simulink library "LM_LIB"  (R2019b)
settings: Solver=VariableStepAuto  StartTime=0.0  StopTime=10.0  RelTol=1e-3
undefined symbols (not defined in the file): P_LM_FusBLParFiltP, P_LM_FusParC0Index, P_LM_FusParC1Index, P_LM_FusParC2Index, P_LM_FusParC3Index, P_LM_OTLBufTPMinPntNum, P_LM_OTLBufTPSPosMinDis, P_LM_OTLRearMaxDis, P_LM_OTLTPNum
libraries: simulink x84, $bdroot x3
(part 2 of 5)

== system LM_LIB/LM_LineInfo1/LM_Line_Fnt ==
  LM_LineC0 : Inport
  LM_PathDisBus : Inport  Port=2
  LM_FusBLInfoFilt : Inport  Port=3
  LM_FusfCamValidInfo : Inport  Port=4
  Bus Selector1 : BusSelector  OutputSignals=LM_FntPath1Dis
  Bus Selector10 : BusSelector  OutputSignals=LM_FusBLFntPath1Info.LM_FusBLPathC0,LM_FusBLFntPath1Info.LM_FusBLPathC1,LM_FusBLFntPath1Info.LM_FusBLPathC2,LM_FusBLFntPath1Info.LM_FusBLPathC3,LM_FusBLFntPath1Info.LM_FusBLPathQuality
  Bus Selector2 : BusSelector  OutputSignals=LM_FntPath1Dis,LM_FntPath2Dis
  Bus Selector3 : BusSelector  OutputSignals=LM_FusBLFntPath2Info.LM_FusBLPathC0,LM_FusBLFntPath2Info.LM_FusBLPathC1,LM_FusBLFntPath2Info.LM_FusBLPathC2,LM_FusBLFntPath2Info.LM_FusBLPathC3,LM_FusBLFntPath2Info.LM_FusBLPathQuality
  Bus Selector5 : BusSelector  OutputSignals=LM_FntPath2Dis,LM_FntPath3Dis
  Bus Selector6 : BusSelector  OutputSignals=LM_FusBLFntPath3Info.LM_FusBLPathC0,LM_FusBLFntPath3Info.LM_FusBLPathC1,LM_FusBLFntPath3Info.LM_FusBLPathC2,LM_FusBLFntPath3Info.LM_FusBLPathC3,LM_FusBLFntPath3Info.LM_FusBLPathQuality
  Bus Selector7 : BusSelector  OutputSignals=LM_FusFntPath1fCamValid
  Bus Selector8 : BusSelector  OutputSignals=LM_FusFntPath2fCamValid
  Bus Selector9 : BusSelector  OutputSignals=LM_FusFntPath3fCamValid
  LM_Path04 : Subsystem
  LM_Path05 : Subsystem
  LM_Path06 : Subsystem
  LM_Path07 : Subsystem
  LM_Path08 : Subsystem
  LM_Line04 : Outport
  LM_Line05 : Outport  Port=2
  LM_LL_Line06 : Outport  Port=3
  LM_LL_Line07 : Outport  Port=4
  LM_LL_Line08 : Outport  Port=5
  wires:
  Bus Selector6/1 -> LM_Path06/2(LM_FusBLFntPath3C0)  "<LM_FusBLPathC0>"
  Bus Selector6/5 -> LM_Path06/6(LM_FusBLFntPath3Quality)  "<LM_FusBLPathQuality>"
  Bus Selector6/4 -> LM_Path06/5(LM_FusBLFntPath3C3)  "<LM_FusBLPathC3>"
  Bus Selector6/3 -> LM_Path06/4(LM_FusBLFntPath3C2)  "<LM_FusBLPathC2>"
  Bus Selector6/2 -> LM_Path06/3(LM_FusBLFntPath3C1)  "<LM_FusBLPathC1>"
  Bus Selector3/1 -> LM_Path05/3(LM_FusBLFntPath2C0)  "<LM_FusBLPathC0>"
  Bus Selector3/5 -> LM_Path05/7(LM_FusBLFntPath2Quality)  "<LM_FusBLPathQuality>"
  Bus Selector3/4 -> LM_Path05/6(LM_FusBLFntPath2C3)  "<LM_FusBLPathC3>"
  Bus Selector3/3 -> LM_Path05/5(LM_FusBLFntPath2C2)  "<LM_FusBLPathC2>"
  Bus Selector3/2 -> LM_Path05/4(LM_FusBLFntPath2C1)  "<LM_FusBLPathC1>"
  Bus Selector10/1 -> LM_Path04/1(LM_FusBLFntPath1C0)  "<LM_FusBLPathC0>"
  Bus Selector10/5 -> LM_Path04/5(LM_FusBLFntPath1Quality)  "<LM_FusBLPathQuality>"
  Bus Selector10/4 -> LM_Path04/4(LM_FusBLFntPath1C3)  "<LM_FusBLPathC3>"
  Bus Selector10/3 -> LM_Path04/3(LM_FusBLFntPath1C2)  "<LM_FusBLPathC2>"
  Bus Selector10/2 -> LM_Path04/2(LM_FusBLFntPath1C1)  "<LM_FusBLPathC1>"
  LM_Path07/1(LM_Line07) -> LM_LL_Line07/1
  LM_Path08/1(LM_Line08) -> LM_LL_Line08/1
  LM_Path06/1(LM_Line06) -> LM_LL_Line06/1
  LM_Path05/1(LM_Line05) -> LM_Line05/1
  LM_Path04/1(LM_Line04) -> LM_Line04/1
  Bus Selector5/2 -> LM_Path06/8(LM_FusBLFntPath3Dis)  "<LM_FntPath3Dis>"
  Bus Selector5/1 -> LM_Path06/7(LM_FusBLFntPath2Dis)  "<LM_FntPath2Dis>"
  LM_LineC0/1 -> LM_Path06/1(LM_LineC0), LM_Path05/8(LM_LineC0), LM_Path04/6(LM_LineC0)
  LM_FusBLInfoFilt/1 -> Bus Selector10/1, Bus Selector6/1, Bus Selector3/1
  Bus Selector2/1 -> LM_Path05/1(LM_FusFntPath1Dis)  "<LM_FntPath1Dis>"
  Bus Selector2/2 -> LM_Path05/2(LM_FusFntPath2Dis)  "<LM_FntPath2Dis>"
  Bus Selector1/1 -> LM_Path04/7(LM_FusFntPath1Dis)  "<LM_FntPath1Dis>"
  LM_PathDisBus/1 -> Bus Selector1/1, Bus Selector5/1, Bus Selector2/1
  LM_FusfCamValidInfo/1 -> Bus Selector7/1, Bus Selector8/1, Bus Selector9/1
  Bus Selector7/1 -> LM_Path04/8(LM_FusFntPath1fCamValid)  "<LM_FusFntPath1fCamValid>"
  Bus Selector8/1 -> LM_Path05/9(LM_FusFntPath2fCamValid)  "<LM_FusFntPath2fCamValid>"
  Bus Selector9/1 -> LM_Path06/9(LM_FusFntPath3fCamValid)  "<LM_FusFntPath3fCamValid>"

== system LM_LIB/LM_LineInfo1/LM_Line_Rear ==
  LM_FusBLInfoFilt : Inport
  LM_PathDisBus : Inport  Port=2
  LM_LineC0 : Inport  Port=3
  Bus Selector1 : BusSelector  OutputSignals=LM_RearPath1Dis
  Bus Selector10 : BusSelector  OutputSignals=LM_RearPath2Dis,LM_RearPath3Dis
  Bus Selector2 : BusSelector  OutputSignals=LM_FusBLRearPath2Info.LM_FusBLPathC0,LM_FusBLRearPath2Info.LM_FusBLPathC1,LM_FusBLRearPath2Info.LM_FusBLPathC2,LM_FusBLRearPath2Info.LM_FusBLPathC3,LM_FusBLRearPath2Info.LM_FusBLPathQuality
  Bus Selector3 : BusSelector  OutputSignals=LM_FusBLRearPath3Info.LM_FusBLPathC0,LM_FusBLRearPath3Info.LM_FusBLPathC1,LM_FusBLRearPath3Info.LM_FusBLPathC2,LM_FusBLRearPath3Info.LM_FusBLPathC3,LM_FusBLRearPath3Info.LM_FusBLPathQuality
  Bus Selector6 : BusSelector  OutputSignals=LM_FusBLRearPath1Info.LM_FusBLPathC0,LM_FusBLRearPath1Info.LM_FusBLPathC1,LM_FusBLRearPath1Info.LM_FusBLPathC2,LM_FusBLRearPath1Info.LM_FusBLPathC3,LM_FusBLRearPath1Info.LM_FusBLPathQuality
  Bus Selector8 : BusSelector  OutputSignals=LM_RearPath1Dis,LM_RearPath2Dis
  LM_Path01 : Subsystem
  LM_Path02 : Subsystem
  LM_Path03 : Subsystem
  LM_Line01 : Outport
  LM_Line02 : Outport  Port=2
  LM_Line03 : Outport  Port=3
  wires:
  Bus Selector10/2 -> LM_Path01/8(LM_RearPath3Dis)  "<LM_RearPath3Dis>"
  Bus Selector10/1 -> LM_Path01/7(LM_RearPath12Dis)  "<LM_RearPath2Dis>"
  Bus Selector3/5 -> LM_Path01/5(LM_FusBLRearPath3Quality)  "<LM_FusBLPathQuality>"
  Bus Selector3/4 -> LM_Path01/4(LM_FusBLRearPath3C3)  "<LM_FusBLPathC3>"
  Bus Selector3/3 -> LM_Path01/3(LM_FusBLRearPath3C2)  "<LM_FusBLPathC2>"
  Bus Selector3/2 -> LM_Path01/2(LM_FusBLRearPath3C1)  "<LM_FusBLPathC1>"
  Bus Selector3/1 -> LM_Path01/1(LM_FusBLRearPath3C0)  "<LM_FusBLPathC0>"
  LM_Path02/1(LM_Line02) -> LM_Line02/1
  Bus Selector8/2 -> LM_Path02/8(LM_RearPath2Dis)  "<LM_RearPath2Dis>"
  Bus Selector8/1 -> LM_Path02/7(LM_RearPath1Dis)  "<LM_RearPath1Dis>"
  Bus Selector2/5 -> LM_Path02/5(LM_FusBLRearPath2Quality)  "<LM_FusBLPathQuality>"
  Bus Selector2/4 -> LM_Path02/4(LM_FusBLRearPath2C3)  "<LM_FusBLPathC3>"
  Bus Selector2/3 -> LM_Path02/3(LM_FusBLRearPath2C2)  "<LM_FusBLPathC2>"
  Bus Selector2/2 -> LM_Path02/2(LM_FusBLRearPath2C1)  "<LM_FusBLPathC1>"
  Bus Selector2/1 -> LM_Path02/1(LM_FusBLRearPath2C0)  "<LM_FusBLPathC0>"
  Bus Selector6/1 -> LM_Path03/1(LM_FusBLRearPath1C0)  "<LM_FusBLPathC0>"
  Bus Selector6/2 -> LM_Path03/2(LM_FusBLRearPath1C1)  "<LM_FusBLPathC1>"
  Bus Selector6/5 -> LM_Path03/5(LM_FusBLRearPath1Quality)  "<LM_FusBLPathQuality>"
  Bus Selector6/3 -> LM_Path03/3(LM_FusBLRearPath1C2)  "<LM_FusBLPathC2>"
  Bus Selector6/4 -> LM_Path03/4(LM_FusBLRearPath1C3)  "<LM_FusBLPathC3>"
  LM_FusBLInfoFilt/1 -> Bus Selector6/1, Bus Selector3/1, Bus Selector2/1
  LM_PathDisBus/1 -> Bus Selector1/1, Bus Selector8/1, Bus Selector10/1
  Bus Selector1/1 -> LM_Path03/7(LM_RearPath1Dis)  "<LM_RearPath1Dis>"
  LM_LineC0/1 -> LM_Path01/6(LM_LineC0), LM_Path02/6(LM_LineC0), LM_Path03/6(LM_LineC0)
  LM_Path03/1(LM_Line03) -> LM_Line03/1
  LM_Path01/1(LM_Line01) -> LM_Line01/1

== system LM_LIB/LM_OTLBuf1InfoNew/LM_OTL_BufLe1InfoUpdate ==
  LM_OTLBufL1DxVectK1Adju : Inport
  LM_OTLBufL1DyVectK1Adju : Inport  Port=2
  LM_OTLBufL1UpdateFlg : Inport  Port=3
  LM_OTLBufL1Objdx : Inport  Port=4
  LM_OTLBufL1Objdy : Inport  Port=5
  LM_OTLBufL1EPPos : Inport  Port=6
  If : If  IfExpression=u1 ~= 0
  If Action Subsystem : Subsystem  TreatAsAtomicUnit=on
  If Action Subsystem1 : Subsystem  TreatAsAtomicUnit=on
  Merge : Merge
  Merge1 : Merge
  LM_OTLBufL1DxVect : Outport  OutDataTypeStr=single  PortDimensions=80
  LM_OTLBufL1DyVect : Outport  Port=2  OutDataTypeStr=single  PortDimensions=80
  wires:
  Merge1/1 -> LM_OTLBufL1DyVect/1  "LM_OTLBufL1DyVect"
  If Action Subsystem1/2(LM_OTLBufL1DyVect) -> Merge1/2
  If Action Subsystem/2(LM_OTLBufL1DyVect) -> Merge1/1
  Merge/1 -> LM_OTLBufL1DxVect/1  "LM_OTLBufL1DxVect"
  If Action Subsystem1/1(LM_OTLBufL1DxVect) -> Merge/2
  If Action Subsystem/1(LM_OTLBufL1DxVect) -> Merge/1
  LM_OTLBufL1EPPos/1 -> If Action Subsystem/3(LM_OTLBufL1EPPos)
  LM_OTLBufL1Objdy/1 -> If Action Subsystem/2(LM_OTLBufL1Objdy)
  LM_OTLBufL1Objdx/1 -> If Action Subsystem/1(LM_OTLBufL1Objdx)
  LM_OTLBufL1DyVectK1Adju/1 -> If Action Subsystem1/2(LM_OTLBufL1DyVectK1Adju), If Action Subsystem/5(LM_OTLBufL1DyVectK1Adju)
  LM_OTLBufL1DxVectK1Adju/1 -> If Action Subsystem1/1(LM_OTLBufL1DxVectK1Adju), If Action Subsystem/4(LM_OTLBufL1DxVectK1Adju)
  If/2 -> If Action Subsystem1/Action
  If/1 -> If Action Subsystem/Action
  LM_OTLBufL1UpdateFlg/1 -> If/1

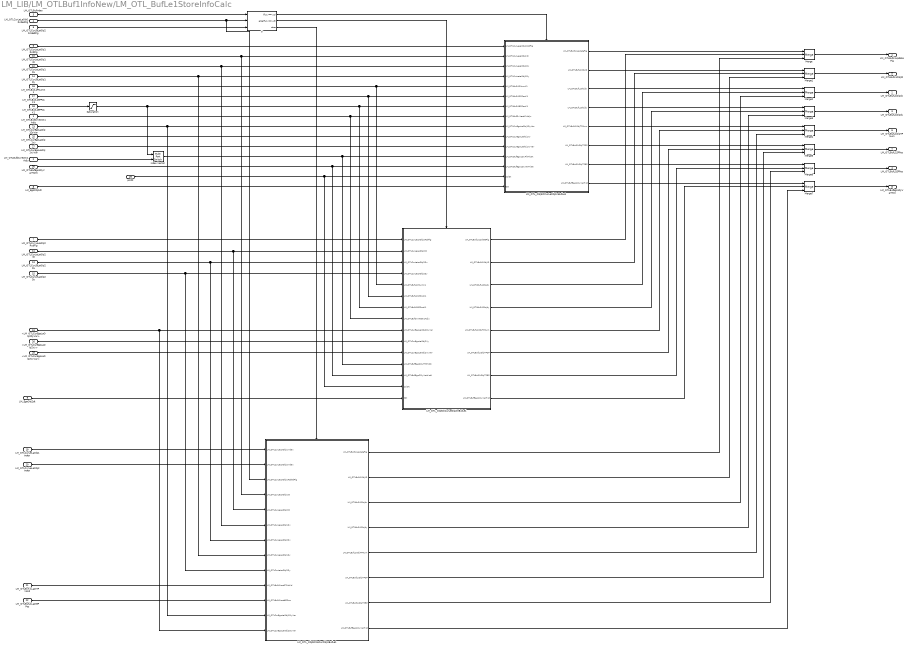
== system LM_LIB/LM_OTLBuf1InfoNew/LM_OTL_BufLe1StoreInfoCalc ==
  LM_OTLBufDxVectK1Adju : Inport
  LM_OTLBufDyVectK1Adju : Inport  Port=2
  LM_OTLBufIndex : Inport  Port=3
  LM_OTLCurLeLaObj1RcdedFlg : Inport  Port=4
  LM_OTLCurLeLaObj2RcdedFlg : Inport  Port=5
  LM_OTLCurLeLaObj1RcdFlg : Inport  Port=6
  LM_OTLCurLeLaObj2RcdFlg : Inport  Port=7
  LM_EgoObj1dt : Inport  Port=8
  LM_EgoObj2dt : Inport  Port=9
  LM_OTLCurLeLaObj1ID : Inport  Port=10
  LM_OTLCurLeLaObj2ID : Inport  Port=11
  LM_OTLCurLeLaObj1Dx : Inport  Port=12
  LM_OTLCurLeLaObj2Dx : Inport  Port=13
  LM_OTLCurLeLaObj1Dy : Inport  Port=14
  LM_OTLCurLeLaObj2Dy : Inport  Port=15
  LM_OTLBufL1PNumK1 : Inport  Port=16
  LM_OTLBufL1SPPosK1 : Inport  Port=17
  LM_OTLBufL1EPPosK1 : Inport  Port=18
  LM_OTLCurLeLaObj1Index : Inport  Port=19
  LM_OTLCurLeLaObj2Index : Inport  Port=20
  LM_OTLBufL1LastTPValid : Inport  Port=21
  LM_OTLBufL1LastEPPos : Inport  Port=22
  LM_OTLCurEgoLaObj1DyVar : Inport  Port=23
  <LM_OTLCurEgoLaObj2DyVar> : Inport  Port=24
  LM_OTLCurEgoLaObj1Vy : Inport  Port=25
  <LM_OTLCurEgoLaObj2Vy> : Inport  Port=26
  LM_OTLCurEgoLaObj1VyVar : Inport  Port=27
  <LM_OTLCurEgoLaObj2VyVar> : Inport  Port=28
  psiDt : Inport  Port=29
  LM_OTLBufEgo1DyVarHistK : Inport  Port=30
  If : If  NumInputs=3  IfExpression=u1 == u2  ElseIfExpressions=u1 == u3
  Index Vector : MultiPortSwitch  Inputs=1
  LM_OTL_ObjSICCurLeObj1InBufLe1 : Subsystem
  LM_OTL_ObjSICCurLeObj2InBufLe1 : Subsystem
  LM_OTL_ObjSICNoCurObjInBufLe1 : Subsystem
  Merge{,1..7} (8 alike) : Merge  Inputs=3
  Saturation : Saturate  UpperLimit=80  LowerLimit=1
  LM_OTLBufL1UpdateFlg : Outport
  LM_OTLBufL1Objdx : Outport  Port=2
  LM_OTLBufL1Objdy : Outport  Port=3
  LM_OTLBufL1EPPos : Outport  Port=4
  LM_OTLBufL1ObjID : Outport  Port=5
  LM_OTLBufL1ObjTPNum : Outport  Port=6
  LM_OTLBufL1SPPos : Outport  Port=7
  LM_OTLBufEgo1DyVarHist : Outport  Port=8
  wires:
  LM_OTLBufIndex/1 -> If/1
  If/1 -> LM_OTL_ObjSICCurLeObj1InBufLe1/Action
  If/2 -> LM_OTL_ObjSICCurLeObj2InBufLe1/Action
  If/3 -> LM_OTL_ObjSICNoCurObjInBufLe1/Action
  LM_OTLCurLeLaObj1RcdedFlg/1 -> If/2, LM_OTL_ObjSICNoCurObjInBufLe1/3(LM_OTLCurLeLaObj1RcdedFlg)
  LM_OTLCurLeLaObj2RcdedFlg/1 -> If/3
  LM_OTLCurLeLaObj1RcdFlg/1 -> LM_OTL_ObjSICCurLeObj1InBufLe1/1(LM_OTLCurLeLaObj1RcdFlg)
  LM_OTLCurLeLaObj1ID/1 -> LM_OTL_ObjSICNoCurObjInBufLe1/4(LM_OTLCurLeLaObj1ID), LM_OTL_ObjSICCurLeObj1InBufLe1/2(LM_OTLCurLeLaObj1ID)
  LM_OTLCurLeLaObj1Dx/1 -> LM_OTL_ObjSICCurLeObj1InBufLe1/3(LM_OTLCurLeLaObj1Dx), LM_OTL_ObjSICNoCurObjInBufLe1/6(LM_OTLCurLeLaObj1Dx)
  LM_OTLCurLeLaObj1Dy/1 -> LM_OTL_ObjSICCurLeObj1InBufLe1/4(LM_OTLCurLeLaObj1Dy), LM_OTL_ObjSICNoCurObjInBufLe1/8(LM_OTLCurLeLaObj1Dy)
  LM_OTLBufL1PNumK1/1 -> LM_OTL_ObjSICCurLeObj2InBufLe1/5(LM_OTLBufL1PNumK1), LM_OTL_ObjSICCurLeObj1InBufLe1/5(LM_OTLBufL1PNumK1)
  LM_OTLBufL1SPPosK1/1 -> LM_OTL_ObjSICCurLeObj2InBufLe1/6(LM_OTLBufL1SPPosK1), LM_OTL_ObjSICCurLeObj1InBufLe1/6(LM_OTLBufL1SPPosK1)
  LM_OTLBufL1EPPosK1/1 -> Saturation/1
  LM_OTLCurLeLaObj2RcdFlg/1 -> LM_OTL_ObjSICCurLeObj2InBufLe1/1(LM_OTLCurLeLaObj2RcdFlg)
  LM_OTLCurLeLaObj2ID/1 -> LM_OTL_ObjSICNoCurObjInBufLe1/5(LM_OTLCurLeLaObj2ID), LM_OTL_ObjSICCurLeObj2InBufLe1/2(LM_OTLCurLeLaObj2ID)
  LM_OTLCurLeLaObj2Dx/1 -> LM_OTL_ObjSICNoCurObjInBufLe1/7(LM_OTLCurLeLaObj2Dx), LM_OTL_ObjSICCurLeObj2InBufLe1/3(LM_OTLCurLeLaObj2Dx)
  LM_OTLCurLeLaObj2Dy/1 -> LM_OTL_ObjSICNoCurObjInBufLe1/9(LM_OTLCurLeLaObj2Dy), LM_OTL_ObjSICCurLeObj2InBufLe1/4(LM_OTLCurLeLaObj2Dy)
  Merge/1 -> LM_OTLBufL1UpdateFlg/1
  Merge1/1 -> LM_OTLBufL1ObjID/1
  Merge2/1 -> LM_OTLBufL1Objdx/1
  Merge3/1 -> LM_OTLBufL1Objdy/1
  Merge4/1 -> LM_OTLBufL1ObjTPNum/1
  Merge5/1 -> LM_OTLBufL1SPPos/1
  LM_OTLCurLeLaObj1Index/1 -> LM_OTL_ObjSICNoCurObjInBufLe1/1(LM_OTLCurLeLaObj1Index)
  LM_OTLCurLeLaObj2Index/1 -> LM_OTL_ObjSICNoCurObjInBufLe1/2(LM_OTLCurLeLaObj2Index)
  LM_OTLBufL1LastTPValid/1 -> LM_OTL_ObjSICNoCurObjInBufLe1/10(LM_OTLBufL1LastTPValid)
  LM_OTLBufL1LastEPPos/1 -> LM_OTL_ObjSICNoCurObjInBufLe1/11(LM_OTLBufL1LastEPPos)
  LM_OTLBufDxVectK1Adju/1 -> LM_OTL_ObjSICCurLeObj2InBufLe1/8(LM_OTLBufDxVectK1Adju), LM_OTL_ObjSICCurLeObj1InBufLe1/8(LM_OTLBufDxVectK1Adju)
  LM_OTLCurEgoLaObj1DyVar/1 -> LM_OTL_ObjSICCurLeObj1InBufLe1/9(LM_OTLCurEgoLaObj1DyVar), LM_OTL_ObjSICNoCurObjInBufLe1/12(LM_OTLCurEgoLaObj1DyVar)
  LM_OTLCurEgoLaObj1Vy/1 -> LM_OTL_ObjSICCurLeObj1InBufLe1/10(LM_OTLCurEgoLaObj1Vy)
  LM_OTLCurEgoLaObj1VyVar/1 -> LM_OTL_ObjSICCurLeObj1InBufLe1/11(LM_OTLCurEgoLaObj1VyVar)
  LM_OTLBufEgo1DyVarHistK/1 -> LM_OTL_ObjSICCurLeObj2InBufLe1/13(LM_OTLBufEgo2DyVarHistK), LM_OTL_ObjSICCurLeObj1InBufLe1/13(LM_OTLBufEgo1DyVarHistK)
  LM_OTLBufDyVectK1Adju/1 -> Index Vector/2
  Index Vector/1 -> LM_OTL_ObjSICCurLeObj2InBufLe1/12(LM_OTLBufEgo2DyFiltHistK), LM_OTL_ObjSICCurLeObj1InBufLe1/12(LM_OTLBufEgo1DyFiltHistK)
  LM_EgoObj1dt/1 -> LM_OTL_ObjSICCurLeObj1InBufLe1/15(tDt)
  psiDt/1 -> LM_OTL_ObjSICCurLeObj2InBufLe1/14(psiDt), LM_OTL_ObjSICCurLeObj1InBufLe1/14(psiDt)
  LM_EgoObj2dt/1 -> LM_OTL_ObjSICCurLeObj2InBufLe1/15(tDt)
  <LM_OTLCurEgoLaObj2DyVar>/1 -> LM_OTL_ObjSICNoCurObjInBufLe1/13(LM_OTLCurEgoLaObj2DyVar), LM_OTL_ObjSICCurLeObj2InBufLe1/9(LM_OTLCurEgoLaObj2DyVar)
  <LM_OTLCurEgoLaObj2Vy>/1 -> LM_OTL_ObjSICCurLeObj2InBufLe1/10(LM_OTLCurEgoLaObj2Vy)
  <LM_OTLCurEgoLaObj2VyVar>/1 -> LM_OTL_ObjSICCurLeObj2InBufLe1/11(LM_OTLCurEgoLaObj2VyVar)
  LM_OTL_ObjSICCurLeObj1InBufLe1/2(LM_OTLBufL1ObjID) -> Merge1/1
  LM_OTL_ObjSICCurLeObj1InBufLe1/3(LM_OTLBufL1Objdx) -> Merge2/1
  LM_OTL_ObjSICCurLeObj1InBufLe1/1(LM_OTLBufL1UpdateFlg) -> Merge/1
  LM_OTL_ObjSICCurLeObj1InBufLe1/4(LM_OTLBufL1Objdy) -> Merge3/1
  LM_OTL_ObjSICCurLeObj1InBufLe1/5(LM_OTLBufL1ObjTPNum) -> Merge4/1
  LM_OTL_ObjSICCurLeObj1InBufLe1/6(LM_OTLBufL1ObjTPSP) -> Merge5/1
  LM_OTL_ObjSICCurLeObj1InBufLe1/7(LM_OTLBufL1ObjTPEP) -> Merge6/1
  LM_OTL_ObjSICCurLeObj2InBufLe1/1(LM_OTLBufL1UpdateFlg) -> Merge/2
  LM_OTL_ObjSICCurLeObj2InBufLe1/2(LM_OTLBufL1ObjID) -> Merge1/2
  LM_OTL_ObjSICCurLeObj2InBufLe1/3(LM_OTLBufL1Objdx) -> Merge2/2
  LM_OTL_ObjSICCurLeObj2InBufLe1/4(LM_OTLBufL1Objdy) -> Merge3/2
  LM_OTL_ObjSICCurLeObj2InBufLe1/5(LM_OTLBufL1ObjTPNum) -> Merge4/2
  LM_OTL_ObjSICCurLeObj2InBufLe1/6(LM_OTLBufL1ObjTPSP) -> Merge5/2
  LM_OTL_ObjSICCurLeObj2InBufLe1/7(LM_OTLBufL1ObjTPEP) -> Merge6/2
  LM_OTL_ObjSICCurLeObj1InBufLe1/8(LM_OTLBufEgo1DyVarHist) -> Merge7/1
  Merge6/1 -> LM_OTLBufL1EPPos/1
  Merge7/1 -> LM_OTLBufEgo1DyVarHist/1
  LM_OTL_ObjSICCurLeObj2InBufLe1/8(LM_OTLBufEgo1DyVarHist) -> Merge7/2
  LM_OTL_ObjSICNoCurObjInBufLe1/1(LM_OTLBufL1UpdateFlg) -> Merge/3
  LM_OTL_ObjSICNoCurObjInBufLe1/2(LM_OTLBufL1ObjID) -> Merge1/3
  LM_OTL_ObjSICNoCurObjInBufLe1/3(LM_OTLBufL1Objdx) -> Merge2/3
  LM_OTL_ObjSICNoCurObjInBufLe1/4(LM_OTLBufL1Objdy) -> Merge3/3
  LM_OTL_ObjSICNoCurObjInBufLe1/5(LM_OTLBufL1ObjTPNum) -> Merge4/3
  LM_OTL_ObjSICNoCurObjInBufLe1/6(LM_OTLBufL1ObjTPSP) -> Merge5/3
  LM_OTL_ObjSICNoCurObjInBufLe1/7(LM_OTLBufL1ObjTPEP) -> Merge6/3
  LM_OTL_ObjSICNoCurObjInBufLe1/8(LM_OTLBufEgo1DyVarHist) -> Merge7/3
  Saturation/1 -> LM_OTL_ObjSICCurLeObj2InBufLe1/7(LM_OTLBufL1EPPosK1), LM_OTL_ObjSICCurLeObj1InBufLe1/7(LM_OTLBufL1EPPosK1), Index Vector/1

== system LM_LIB/LM_OTLBuf2InfoNew/LM_OTL_BufLe1InfoUpdate ==
  LM_OTLBufL1DxVectK1Adju : Inport
  LM_OTLBufL1DyVectK1Adju : Inport  Port=2
  LM_OTLBufL1UpdateFlg : Inport  Port=3
  LM_OTLBufL1Objdx : Inport  Port=4
  LM_OTLBufL1Objdy : Inport  Port=5
  LM_OTLBufL1EPPos : Inport  Port=6
  If : If  IfExpression=u1 ~= 0
  If Action Subsystem : Subsystem  TreatAsAtomicUnit=on
  If Action Subsystem1 : Subsystem  TreatAsAtomicUnit=on
  Merge : Merge
  Merge1 : Merge
  LM_OTLBufL1DxVect : Outport  OutDataTypeStr=single  PortDimensions=80
  LM_OTLBufL1DyVect : Outport  Port=2  OutDataTypeStr=single  PortDimensions=80
  wires:
  Merge1/1 -> LM_OTLBufL1DyVect/1  "LM_OTLBufL1DyVect"
  If Action Subsystem1/2(LM_OTLBufL1DyVect) -> Merge1/2
  If Action Subsystem/2(LM_OTLBufL1DyVect) -> Merge1/1
  Merge/1 -> LM_OTLBufL1DxVect/1  "LM_OTLBufL1DxVect"
  If Action Subsystem1/1(LM_OTLBufL1DxVect) -> Merge/2
  If Action Subsystem/1(LM_OTLBufL1DxVect) -> Merge/1
  LM_OTLBufL1EPPos/1 -> If Action Subsystem/3(LM_OTLBufL1EPPos)
  LM_OTLBufL1Objdy/1 -> If Action Subsystem/2(LM_OTLBufL1Objdy)
  LM_OTLBufL1Objdx/1 -> If Action Subsystem/1(LM_OTLBufL1Objdx)
  LM_OTLBufL1DyVectK1Adju/1 -> If Action Subsystem1/2(LM_OTLBufL1DyVectK1Adju), If Action Subsystem/5(LM_OTLBufL1DyVectK1Adju)
  LM_OTLBufL1DxVectK1Adju/1 -> If Action Subsystem1/1(LM_OTLBufL1DxVectK1Adju), If Action Subsystem/4(LM_OTLBufL1DxVectK1Adju)
  If/2 -> If Action Subsystem1/Action
  If/1 -> If Action Subsystem/Action
  LM_OTLBufL1UpdateFlg/1 -> If/1

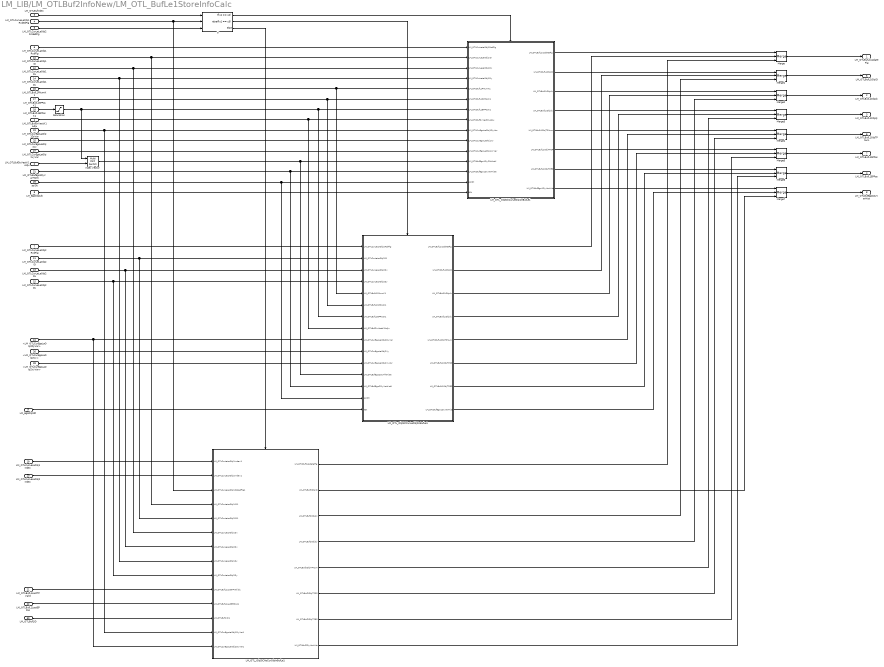
== system LM_LIB/LM_OTLBuf2InfoNew/LM_OTL_BufLe1StoreInfoCalc ==
  LM_OTLBufDxVectK1Adju : Inport
  LM_OTLBufDyVectK1Adju : Inport  Port=2
  LM_OTLBufIndex : Inport  Port=3
  LM_OTLCurLeLaObj1RcdedFlg : Inport  Port=4
  LM_OTLCurLeLaObj2RcdedFlg : Inport  Port=5
  LM_OTLCurLeLaObj1RcdFlg : Inport  Port=6
  LM_OTLCurLeLaObj2RcdFlg : Inport  Port=7
  LM_EgoObj1dt : Inport  Port=8
  LM_EgoObj2dt : Inport  Port=9
  LM_OTLCurLeLaObj1ID : Inport  Port=10
  LM_OTLCurLeLaObj2ID : Inport  Port=11
  LM_OTLCurLeLaObj1Dx : Inport  Port=12
  LM_OTLCurLeLaObj2Dx : Inport  Port=13
  LM_OTLCurLeLaObj1Dy : Inport  Port=14
  LM_OTLCurLeLaObj2Dy : Inport  Port=15
  LM_OTLBufL1PNumK1 : Inport  Port=16
  LM_OTLBufL1SPPosK1 : Inport  Port=17
  LM_OTLBufL1EPPosK1 : Inport  Port=18
  LM_OTLCurLeLaObj1Index : Inport  Port=19
  LM_OTLCurLeLaObj2Index : Inport  Port=20
  LM_OTLBufL1LastTPValid : Inport  Port=21
  LM_OTLBufL1LastEPPos : Inport  Port=22
  LM_OTLCurEgoLaObj1DyVar : Inport  Port=23
  <LM_OTLCurEgoLaObj2DyVar> : Inport  Port=24
  LM_OTLCurEgoLaObj1Vy : Inport  Port=25
  <LM_OTLCurEgoLaObj2Vy> : Inport  Port=26
  LM_OTLCurEgoLaObj1VyVar : Inport  Port=27
  <LM_OTLCurEgoLaObj2VyVar> : Inport  Port=28
  psiDt : Inport  Port=29
  LM_OTLBuf1ID : Inport  Port=30
  LM_OTLBufEgo1DyVarHistK : Inport  Port=31
  If : If  NumInputs=3  IfExpression=u1 == u2  ElseIfExpressions=u1 == u3
  Index Vector : MultiPortSwitch  Inputs=1
  LM_OTL_ObjSICCurLeObj1InBufLe1 : Subsystem
  LM_OTL_ObjSICCurLeObj2InBufLe1 : Subsystem
  LM_OTL_ObjSICNoCurObjInBufLe1 : Subsystem
  Merge{,1..7} (8 alike) : Merge  Inputs=3
  Saturation : Saturate  UpperLimit=80  LowerLimit=1
  LM_OTLBufL1UpdateFlg : Outport
  LM_OTLBufL1Objdx : Outport  Port=2
  LM_OTLBufL1Objdy : Outport  Port=3
  LM_OTLBufL1EPPos : Outport  Port=4
  LM_OTLBufL1ObjID : Outport  Port=5
  LM_OTLBufL1ObjTPNum : Outport  Port=6
  LM_OTLBufL1SPPos : Outport  Port=7
  LM_OTLBufEgo1DyVarHist : Outport  Port=8
  wires:
  LM_OTLBufIndex/1 -> If/1
  If/1 -> LM_OTL_ObjSICCurLeObj1InBufLe1/Action
  If/2 -> LM_OTL_ObjSICCurLeObj2InBufLe1/Action
  If/3 -> LM_OTL_ObjSICNoCurObjInBufLe1/Action
  LM_OTLCurLeLaObj1RcdedFlg/1 -> LM_OTL_ObjSICNoCurObjInBufLe1/3(LM_OTLCurLeLaObj1RcdedFlg1), If/2
  LM_OTLCurLeLaObj2RcdedFlg/1 -> If/3
  LM_OTLCurLeLaObj1RcdFlg/1 -> LM_OTL_ObjSICCurLeObj1InBufLe1/1(LM_OTLCurLeLaObj1RcdFlg)
  LM_OTLCurLeLaObj1ID/1 -> LM_OTL_ObjSICNoCurObjInBufLe1/4(LM_OTLCurLeLaObj1ID1), LM_OTL_ObjSICCurLeObj1InBufLe1/2(LM_OTLCurLeLaObj1ID)
  LM_OTLCurLeLaObj1Dy/1 -> LM_OTL_ObjSICNoCurObjInBufLe1/8(LM_OTLCurLeLaObj1Dy), LM_OTL_ObjSICCurLeObj1InBufLe1/4(LM_OTLCurLeLaObj1Dy)
  LM_OTLBufL1PNumK1/1 -> LM_OTL_ObjSICCurLeObj2InBufLe1/5(LM_OTLBufL1PNumK1), LM_OTL_ObjSICCurLeObj1InBufLe1/5(LM_OTLBufL1PNumK1)
  LM_OTLBufL1SPPosK1/1 -> LM_OTL_ObjSICCurLeObj2InBufLe1/6(LM_OTLBufL1SPPosK1), LM_OTL_ObjSICCurLeObj1InBufLe1/6(LM_OTLBufL1SPPosK1)
  LM_OTLBufL1EPPosK1/1 -> Saturation/1
  LM_OTLCurLeLaObj2RcdFlg/1 -> LM_OTL_ObjSICCurLeObj2InBufLe1/1(LM_OTLCurLeLaObj2RcdFlg)
  LM_OTLCurLeLaObj2ID/1 -> LM_OTL_ObjSICNoCurObjInBufLe1/5(LM_OTLCurLeLaObj2ID1), LM_OTL_ObjSICCurLeObj2InBufLe1/2(LM_OTLCurLeLaObj2ID)
  LM_OTLCurLeLaObj2Dx/1 -> LM_OTL_ObjSICNoCurObjInBufLe1/7(LM_OTLCurLeLaObj2Dx), LM_OTL_ObjSICCurLeObj2InBufLe1/3(LM_OTLCurLeLaObj2Dx)
  LM_OTLCurLeLaObj2Dy/1 -> LM_OTL_ObjSICNoCurObjInBufLe1/9(LM_OTLCurLeLaObj2Dy), LM_OTL_ObjSICCurLeObj2InBufLe1/4(LM_OTLCurLeLaObj2Dy)
  Merge/1 -> LM_OTLBufL1UpdateFlg/1
  Merge1/1 -> LM_OTLBufL1ObjID/1
  Merge2/1 -> LM_OTLBufL1Objdx/1
  Merge3/1 -> LM_OTLBufL1Objdy/1
  Merge4/1 -> LM_OTLBufL1ObjTPNum/1
  Merge5/1 -> LM_OTLBufL1SPPos/1
  LM_OTLBufDxVectK1Adju/1 -> LM_OTL_ObjSICCurLeObj2InBufLe1/8(LM_OTLBufDxVectK1Adju), LM_OTL_ObjSICCurLeObj1InBufLe1/8(LM_OTLBufDxVectK1Adju)
  LM_OTLCurEgoLaObj1DyVar/1 -> LM_OTL_ObjSICCurLeObj1InBufLe1/9(LM_OTLCurEgoLaObj1DyVar), LM_OTL_ObjSICNoCurObjInBufLe1/13(LM_OTLCurEgoLaObj1DyVar1)
  LM_OTLCurEgoLaObj1Vy/1 -> LM_OTL_ObjSICCurLeObj1InBufLe1/10(LM_OTLCurEgoLaObj1Vy)
  LM_OTLCurEgoLaObj1VyVar/1 -> LM_OTL_ObjSICCurLeObj1InBufLe1/11(LM_OTLCurEgoLaObj1VyVar)
  LM_OTLBufEgo1DyVarHistK/1 -> LM_OTL_ObjSICCurLeObj2InBufLe1/13(LM_OTLBufEgo2DyVarHistK), LM_OTL_ObjSICCurLeObj1InBufLe1/13(LM_OTLBufEgo1DyVarHistK)
  LM_OTLBufDyVectK1Adju/1 -> Index Vector/2
  Index Vector/1 -> LM_OTL_ObjSICCurLeObj2InBufLe1/12(LM_OTLBufEgo2DyFiltHistK), LM_OTL_ObjSICCurLeObj1InBufLe1/12(LM_OTLBufEgo1DyFiltHistK)
  LM_EgoObj1dt/1 -> LM_OTL_ObjSICCurLeObj1InBufLe1/15(tDt)
  psiDt/1 -> LM_OTL_ObjSICCurLeObj2InBufLe1/14(psiDt), LM_OTL_ObjSICCurLeObj1InBufLe1/14(psiDt)
  LM_EgoObj2dt/1 -> LM_OTL_ObjSICCurLeObj2InBufLe1/15(tDt)
  <LM_OTLCurEgoLaObj2DyVar>/1 -> LM_OTL_ObjSICCurLeObj2InBufLe1/9(LM_OTLCurEgoLaObj2DyVar), LM_OTL_ObjSICNoCurObjInBufLe1/14(LM_OTLCurEgoLaObj2DyVar1)
  <LM_OTLCurEgoLaObj2Vy>/1 -> LM_OTL_ObjSICCurLeObj2InBufLe1/10(LM_OTLCurEgoLaObj2Vy)
  <LM_OTLCurEgoLaObj2VyVar>/1 -> LM_OTL_ObjSICCurLeObj2InBufLe1/11(LM_OTLCurEgoLaObj2VyVar)
  LM_OTL_ObjSICCurLeObj1InBufLe1/2(LM_OTLBufL1ObjID) -> Merge1/1
  LM_OTL_ObjSICCurLeObj1InBufLe1/3(LM_OTLBufL1Objdx) -> Merge2/1
  LM_OTL_ObjSICCurLeObj1InBufLe1/1(LM_OTLBufL1UpdateFlg) -> Merge/1
  LM_OTL_ObjSICCurLeObj1InBufLe1/4(LM_OTLBufL1Objdy) -> Merge3/1
  LM_OTL_ObjSICCurLeObj1InBufLe1/5(LM_OTLBufL1ObjTPNum) -> Merge4/1
  LM_OTL_ObjSICCurLeObj1InBufLe1/6(LM_OTLBufL1ObjTPSP) -> Merge5/1
  LM_OTL_ObjSICCurLeObj1InBufLe1/7(LM_OTLBufL1ObjTPEP) -> Merge6/1
  LM_OTL_ObjSICCurLeObj2InBufLe1/1(LM_OTLBufL1UpdateFlg) -> Merge/2
  LM_OTL_ObjSICCurLeObj2InBufLe1/2(LM_OTLBufL1ObjID) -> Merge1/2
  LM_OTL_ObjSICCurLeObj2InBufLe1/3(LM_OTLBufL1Objdx) -> Merge2/2
  LM_OTL_ObjSICCurLeObj2InBufLe1/4(LM_OTLBufL1Objdy) -> Merge3/2
  LM_OTL_ObjSICCurLeObj2InBufLe1/5(LM_OTLBufL1ObjTPNum) -> Merge4/2
  LM_OTL_ObjSICCurLeObj2InBufLe1/6(LM_OTLBufL1ObjTPSP) -> Merge5/2
  LM_OTL_ObjSICCurLeObj2InBufLe1/7(LM_OTLBufL1ObjTPEP) -> Merge6/2
  LM_OTL_ObjSICCurLeObj1InBufLe1/8(LM_OTLBufEgo1DyVarHist) -> Merge7/1
  Merge6/1 -> LM_OTLBufL1EPPos/1
  Merge7/1 -> LM_OTLBufEgo1DyVarHist/1
  LM_OTL_ObjSICCurLeObj2InBufLe1/8(LM_OTLBufEgo1DyVarHist) -> Merge7/2
  LM_OTL_ObjSICNoCurObjInBufLe1/1(LM_OTLBuf2UpdateFlg) -> Merge/3
  LM_OTL_ObjSICNoCurObjInBufLe1/3(LM_OTLBuf2Objdx) -> Merge1/3
  LM_OTL_ObjSICNoCurObjInBufLe1/4(LM_OTLBuf2Objdy) -> Merge2/3
  LM_OTL_ObjSICNoCurObjInBufLe1/5(LM_OTLBuf2ObjTPNum) -> Merge3/3
  LM_OTL_ObjSICNoCurObjInBufLe1/6(LM_OTLBuf2ObjTPSP) -> Merge4/3
  LM_OTL_ObjSICNoCurObjInBufLe1/7(LM_OTLBuf2ObjTPEP) -> Merge5/3
  LM_OTL_ObjSICNoCurObjInBufLe1/8(LM_OTLBuf2DyVarHist) -> Merge6/3
  LM_OTL_ObjSICNoCurObjInBufLe1/2(LM_OTLBuf2ObjID) -> Merge7/3
  LM_OTLCurLeLaObj1Index/1 -> LM_OTL_ObjSICNoCurObjInBufLe1/1(LM_OTLCurLeLaObj1Index1)
  LM_OTLCurLeLaObj2Index/1 -> LM_OTL_ObjSICNoCurObjInBufLe1/2(LM_OTLCurLeLaObj2Index1)
  LM_OTLCurLeLaObj1Dx/1 -> LM_OTL_ObjSICNoCurObjInBufLe1/6(LM_OTLCurLeLaObj1Dx), LM_OTL_ObjSICCurLeObj1InBufLe1/3(LM_OTLCurLeLaObj1Dx)
  LM_OTLBufL1LastTPValid/1 -> LM_OTL_ObjSICNoCurObjInBufLe1/10(LM_OTLBufL1LastTPValid1)
  LM_OTLBufL1LastEPPos/1 -> LM_OTL_ObjSICNoCurObjInBufLe1/11(LM_OTLBufL1LastEPPos1)
  LM_OTLBuf1ID/1 -> LM_OTL_ObjSICNoCurObjInBufLe1/12(LM_OTLBuf1ID1)
  Saturation/1 -> LM_OTL_ObjSICCurLeObj2InBufLe1/7(LM_OTLBufL1EPPosK1), LM_OTL_ObjSICCurLeObj1InBufLe1/7(LM_OTLBufL1EPPosK1), Index Vector/1

== system LM_LIB/LM_OTLBufLostTPValidJudgeNew/If Action Subsystem ==
  LM_OTLBufL1DxVectK1Adju : Inport
  LM_OTLBufPNumK1 : Inport  Port=2
  LM_OTLBufSPPosK1 : Inport  Port=3
  LM_OTLBufEPPosK1 : Inport  Port=4
  LM_OTLBufLastTPValidK1 : Inport  Port=5
  LM_OTLBufLastPNumK1 : Inport  Port=6
  LM_OTLBufLastSPPosK1 : Inport  Port=7
  LM_OTLBufLastEPPosK1 : Inport  Port=8
  Action Port : ActionPort  ActionPortLabel=if(u1 > 0)
  If : If  IfExpression=u1 ~= 0
  If Action Subsystem : Subsystem  TreatAsAtomicUnit=on
  If Action Subsystem1 : Subsystem  TreatAsAtomicUnit=on
  Merge{,1..3} (4 alike) : Merge
  LM_OTLBufLastTPValid : Outport
  LM_OTLBufLastPNum : Outport  Port=2
  LM_OTLBufLastSPPos : Outport  Port=3
  LM_OTLBufLastEPPos : Outport  Port=4
  wires:
  LM_OTLBufLastTPValidK1/1 -> If/1
  If/1 -> If Action Subsystem/Action
  If/2 -> If Action Subsystem1/Action
  LM_OTLBufL1DxVectK1Adju/1 -> If Action Subsystem1/1(LM_OTLBufL1DxVectK1Adju), If Action Subsystem/4(LM_OTLBufL1DxVectK1Adju)
  LM_OTLBufPNumK1/1 -> If Action Subsystem1/2(LM_OTLBufPNumK1), If Action Subsystem/5(LM_OTLBufPNumK1)
  LM_OTLBufSPPosK1/1 -> If Action Subsystem/6(LM_OTLBufSPPosK1), If Action Subsystem1/3(LM_OTLBufSPPosK1)
  LM_OTLBufEPPosK1/1 -> If Action Subsystem/7(LM_OTLBufEPPosK1), If Action Subsystem1/4(LM_OTLBufEPPosK1)
  LM_OTLBufLastSPPosK1/1 -> If Action Subsystem/2(LM_OTLBufLastSPPosK1)
  LM_OTLBufLastPNumK1/1 -> If Action Subsystem/1(LM_OTLBufLastPNumK1)
  LM_OTLBufLastEPPosK1/1 -> If Action Subsystem/3(LM_OTLBufLastEPPosK1)
  Merge3/1 -> LM_OTLBufLastEPPos/1  "LM_OTLBufLastEPPos"
  Merge2/1 -> LM_OTLBufLastSPPos/1  "LM_OTLBufLastSPPos"
  Merge1/1 -> LM_OTLBufLastPNum/1  "LM_OTLBufLastPNum"
  Merge/1 -> LM_OTLBufLastTPValid/1  "LM_OTLBufLastTPValid"
  If Action Subsystem/1(LM_OTLBufLastTPValid) -> Merge/1
  If Action Subsystem1/1(LM_OTLBufLastTPValid) -> Merge/2
  If Action Subsystem/2(LM_OTLBufLastPNum) -> Merge1/1
  If Action Subsystem1/2(LM_OTLBufLastPNum) -> Merge1/2
  If Action Subsystem/3(LM_OTLBufLastSPPos) -> Merge2/1
  If Action Subsystem/4(LM_OTLBufLastEPPos) -> Merge3/1
  If Action Subsystem1/3(LM_OTLBufLastSPPos) -> Merge2/2
  If Action Subsystem1/4(LM_OTLBufLastEPPos) -> Merge3/2

== system LM_LIB/LM_OTLBufLostTPValidJudgeNew/If Action Subsystem1 ==
  LM_OTLBufLastTPValidK1 : Inport
  LM_OTLBufLastPNumK1 : Inport  Port=2
  LM_OTLBufLastSPPosK1 : Inport  Port=3
  LM_OTLBufLastEPPosK1 : Inport  Port=4
  Action Port : ActionPort  ActionPortLabel=else
  LM_OTLBufLastTPValid : Outport
  LM_OTLBufLastPNum : Outport  Port=2
  LM_OTLBufLastSPPos : Outport  Port=3
  LM_OTLBufLastEPPos : Outport  Port=4
  wires:
  LM_OTLBufLastTPValidK1/1 -> LM_OTLBufLastTPValid/1  "LM_OTLBufLastTPValid"
  LM_OTLBufLastPNumK1/1 -> LM_OTLBufLastPNum/1  "LM_OTLBufLastPNum"
  LM_OTLBufLastSPPosK1/1 -> LM_OTLBufLastSPPos/1  "LM_OTLBufLastSPPos"
  LM_OTLBufLastEPPosK1/1 -> LM_OTLBufLastEPPos/1  "LM_OTLBufLastEPPos"

== system LM_LIB/LM_OTL_Buf1InfoUpdate/LM_OTL_BufLe1InfoUpdate ==
  LM_OTLBufL1DxVectK1Adju : Inport
  LM_OTLBufL1DyVectK1Adju : Inport  Port=2
  LM_OTLBufL1UpdateFlg : Inport  Port=3
  LM_OTLBufL1Objdx : Inport  Port=4
  LM_OTLBufL1Objdy : Inport  Port=5
  LM_OTLBufL1EPPos : Inport  Port=6
  If : If  IfExpression=u1 ~= 0
  If Action Subsystem : Subsystem  TreatAsAtomicUnit=on
  If Action Subsystem1 : Subsystem  TreatAsAtomicUnit=on
  Merge : Merge
  Merge1 : Merge
  LM_OTLBufL1DxVect : Outport  OutDataTypeStr=single  PortDimensions=80
  LM_OTLBufL1DyVect : Outport  Port=2  OutDataTypeStr=single  PortDimensions=80
  wires:
  Merge1/1 -> LM_OTLBufL1DyVect/1  "LM_OTLBufL1DyVect"
  If Action Subsystem1/2(LM_OTLBufL1DyVect) -> Merge1/2
  If Action Subsystem/2(LM_OTLBufL1DyVect) -> Merge1/1
  Merge/1 -> LM_OTLBufL1DxVect/1  "LM_OTLBufL1DxVect"
  If Action Subsystem1/1(LM_OTLBufL1DxVect) -> Merge/2
  If Action Subsystem/1(LM_OTLBufL1DxVect) -> Merge/1
  LM_OTLBufL1EPPos/1 -> If Action Subsystem/3(LM_OTLBufL1EPPos)
  LM_OTLBufL1Objdy/1 -> If Action Subsystem/2(LM_OTLBufL1Objdy)
  LM_OTLBufL1Objdx/1 -> If Action Subsystem/1(LM_OTLBufL1Objdx)
  LM_OTLBufL1DyVectK1Adju/1 -> If Action Subsystem1/2(LM_OTLBufL1DyVectK1Adju), If Action Subsystem/5(LM_OTLBufL1DyVectK1Adju)
  LM_OTLBufL1DxVectK1Adju/1 -> If Action Subsystem1/1(LM_OTLBufL1DxVectK1Adju), If Action Subsystem/4(LM_OTLBufL1DxVectK1Adju)
  If/2 -> If Action Subsystem1/Action
  If/1 -> If Action Subsystem/Action
  LM_OTLBufL1UpdateFlg/1 -> If/1

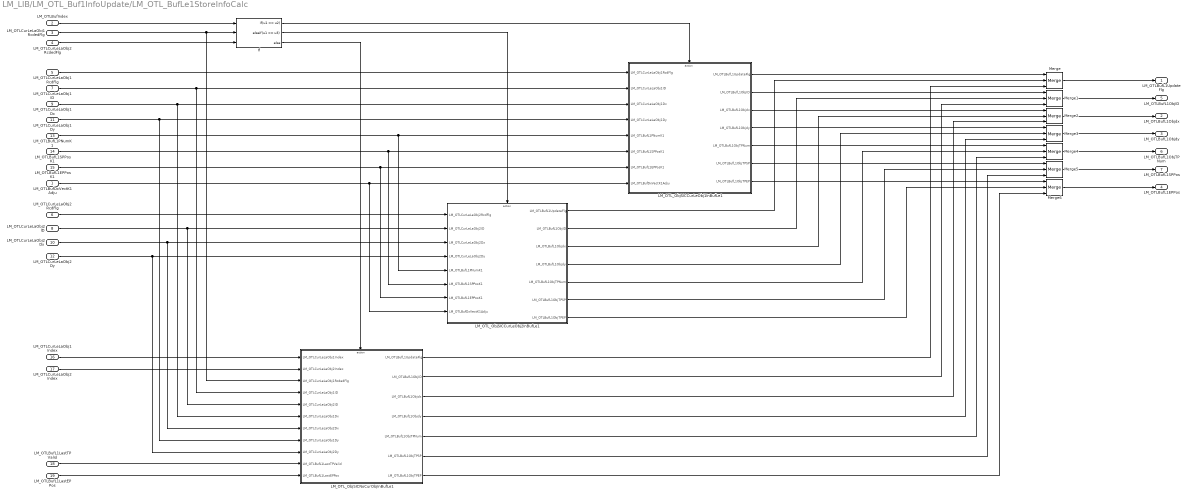
== system LM_LIB/LM_OTL_Buf1InfoUpdate/LM_OTL_BufLe1StoreInfoCalc ==
  LM_OTLBufDxVectK1Adju : Inport
  LM_OTLBufIndex : Inport  Port=2
  LM_OTLCurLeLaObj1RcdedFlg : Inport  Port=3
  LM_OTLCurLeLaObj2RcdedFlg : Inport  Port=4
  LM_OTLCurLeLaObj1RcdFlg : Inport  Port=5
  LM_OTLCurLeLaObj2RcdFlg : Inport  Port=6
  LM_OTLCurLeLaObj1ID : Inport  Port=7
  LM_OTLCurLeLaObj2ID : Inport  Port=8
  LM_OTLCurLeLaObj1Dx : Inport  Port=9
  LM_OTLCurLeLaObj2Dx : Inport  Port=10
  LM_OTLCurLeLaObj1Dy : Inport  Port=11
  LM_OTLCurLeLaObj2Dy : Inport  Port=12
  LM_OTLBufL1PNumK1 : Inport  Port=13
  LM_OTLBufL1SPPosK1 : Inport  Port=14
  LM_OTLBufL1EPPosK1 : Inport  Port=15
  LM_OTLCurLeLaObj1Index : Inport  Port=16
  LM_OTLCurLeLaObj2Index : Inport  Port=17
  LM_OTLBufL1LastTPValid : Inport  Port=18
  LM_OTLBufL1LastEPPos : Inport  Port=19
  If : If  NumInputs=3  IfExpression=u1 == u2  ElseIfExpressions=u1 == u3
  LM_OTL_ObjSICCurLeObj1InBufLe1 : Subsystem
  LM_OTL_ObjSICCurLeObj2InBufLe1 : Subsystem
  LM_OTL_ObjSICNoCurObjInBufLe1 : Subsystem
  Merge{,1..6} (7 alike) : Merge  Inputs=3
  LM_OTLBufL1UpdateFlg : Outport
  LM_OTLBufL1Objdx : Outport  Port=2
  LM_OTLBufL1Objdy : Outport  Port=3
  LM_OTLBufL1EPPos : Outport  Port=4
  LM_OTLBufL1ObjID : Outport  Port=5
  LM_OTLBufL1ObjTPNum : Outport  Port=6
  LM_OTLBufL1SPPos : Outport  Port=7
  wires:
  LM_OTLBufIndex/1 -> If/1
  If/1 -> LM_OTL_ObjSICCurLeObj1InBufLe1/Action
  If/2 -> LM_OTL_ObjSICCurLeObj2InBufLe1/Action
  If/3 -> LM_OTL_ObjSICNoCurObjInBufLe1/Action
  LM_OTLCurLeLaObj1RcdedFlg/1 -> LM_OTL_ObjSICNoCurObjInBufLe1/3(LM_OTLCurLeLaObj1RcdedFlg), If/2
  LM_OTLCurLeLaObj2RcdedFlg/1 -> If/3
  LM_OTLCurLeLaObj1RcdFlg/1 -> LM_OTL_ObjSICCurLeObj1InBufLe1/1(LM_OTLCurLeLaObj1RcdFlg)
  LM_OTLCurLeLaObj1ID/1 -> LM_OTL_ObjSICNoCurObjInBufLe1/4(LM_OTLCurLeLaObj1ID), LM_OTL_ObjSICCurLeObj1InBufLe1/2(LM_OTLCurLeLaObj1ID)
  LM_OTLCurLeLaObj1Dx/1 -> LM_OTL_ObjSICNoCurObjInBufLe1/6(LM_OTLCurLeLaObj1Dx), LM_OTL_ObjSICCurLeObj1InBufLe1/3(LM_OTLCurLeLaObj1Dx)
  LM_OTLCurLeLaObj1Dy/1 -> LM_OTL_ObjSICNoCurObjInBufLe1/8(LM_OTLCurLeLaObj1Dy), LM_OTL_ObjSICCurLeObj1InBufLe1/4(LM_OTLCurLeLaObj1Dy)
  LM_OTLBufL1PNumK1/1 -> LM_OTL_ObjSICCurLeObj2InBufLe1/5(LM_OTLBufL1PNumK1), LM_OTL_ObjSICCurLeObj1InBufLe1/5(LM_OTLBufL1PNumK1)
  LM_OTLBufL1SPPosK1/1 -> LM_OTL_ObjSICCurLeObj2InBufLe1/6(LM_OTLBufL1SPPosK1), LM_OTL_ObjSICCurLeObj1InBufLe1/6(LM_OTLBufL1SPPosK1)
  LM_OTLBufL1EPPosK1/1 -> LM_OTL_ObjSICCurLeObj2InBufLe1/7(LM_OTLBufL1EPPosK1), LM_OTL_ObjSICCurLeObj1InBufLe1/7(LM_OTLBufL1EPPosK1)
  LM_OTLCurLeLaObj2RcdFlg/1 -> LM_OTL_ObjSICCurLeObj2InBufLe1/1(LM_OTLCurLeLaObj2RcdFlg)
  LM_OTLCurLeLaObj2ID/1 -> LM_OTL_ObjSICNoCurObjInBufLe1/5(LM_OTLCurLeLaObj2ID), LM_OTL_ObjSICCurLeObj2InBufLe1/2(LM_OTLCurLeLaObj2ID)
  LM_OTLCurLeLaObj2Dx/1 -> LM_OTL_ObjSICNoCurObjInBufLe1/7(LM_OTLCurLeLaObj2Dx), LM_OTL_ObjSICCurLeObj2InBufLe1/3(LM_OTLCurLeLaObj2Dx)
  LM_OTLCurLeLaObj2Dy/1 -> LM_OTL_ObjSICNoCurObjInBufLe1/9(LM_OTLCurLeLaObj2Dy), LM_OTL_ObjSICCurLeObj2InBufLe1/4(LM_OTLCurLeLaObj2Dy)
  LM_OTL_ObjSICCurLeObj1InBufLe1/1(LM_OTLBufL1UpdateFlg) -> Merge/1
  Merge/1 -> LM_OTLBufL1UpdateFlg/1
  LM_OTL_ObjSICCurLeObj1InBufLe1/2(LM_OTLBufL1ObjID) -> Merge1/1
  Merge1/1 -> LM_OTLBufL1ObjID/1
  LM_OTL_ObjSICCurLeObj1InBufLe1/3(LM_OTLBufL1Objdx) -> Merge2/1
  Merge2/1 -> LM_OTLBufL1Objdx/1
  LM_OTL_ObjSICCurLeObj1InBufLe1/4(LM_OTLBufL1Objdy) -> Merge3/1
  Merge3/1 -> LM_OTLBufL1Objdy/1
  LM_OTL_ObjSICCurLeObj1InBufLe1/5(LM_OTLBufL1ObjTPNum) -> Merge4/1
  Merge4/1 -> LM_OTLBufL1ObjTPNum/1
  LM_OTL_ObjSICCurLeObj1InBufLe1/6(LM_OTLBufL1ObjTPSP) -> Merge5/1
  Merge5/1 -> LM_OTLBufL1SPPos/1
  LM_OTL_ObjSICCurLeObj1InBufLe1/7(LM_OTLBufL1ObjTPEP) -> Merge6/1
  Merge6/1 -> LM_OTLBufL1EPPos/1
  LM_OTL_ObjSICCurLeObj2InBufLe1/1(LM_OTLBufL1UpdateFlg) -> Merge/2
  LM_OTL_ObjSICCurLeObj2InBufLe1/2(LM_OTLBufL1ObjID) -> Merge1/2
  LM_OTL_ObjSICCurLeObj2InBufLe1/3(LM_OTLBufL1Objdx) -> Merge2/2
  LM_OTL_ObjSICCurLeObj2InBufLe1/4(LM_OTLBufL1Objdy) -> Merge3/2
  LM_OTL_ObjSICCurLeObj2InBufLe1/5(LM_OTLBufL1ObjTPNum) -> Merge4/2
  LM_OTL_ObjSICCurLeObj2InBufLe1/6(LM_OTLBufL1ObjTPSP) -> Merge5/2
  LM_OTL_ObjSICCurLeObj2InBufLe1/7(LM_OTLBufL1ObjTPEP) -> Merge6/2
  LM_OTL_ObjSICNoCurObjInBufLe1/1(LM_OTLBufL1UpdateFlg) -> Merge/3
  LM_OTL_ObjSICNoCurObjInBufLe1/2(LM_OTLBufL1ObjID) -> Merge1/3
  LM_OTL_ObjSICNoCurObjInBufLe1/3(LM_OTLBufL1Objdx) -> Merge2/3
  LM_OTL_ObjSICNoCurObjInBufLe1/4(LM_OTLBufL1Objdy) -> Merge3/3
  LM_OTL_ObjSICNoCurObjInBufLe1/5(LM_OTLBufL1ObjTPNum) -> Merge4/3
  LM_OTL_ObjSICNoCurObjInBufLe1/6(LM_OTLBufL1ObjTPSP) -> Merge5/3
  LM_OTL_ObjSICNoCurObjInBufLe1/7(LM_OTLBufL1ObjTPEP) -> Merge6/3
  LM_OTLCurLeLaObj1Index/1 -> LM_OTL_ObjSICNoCurObjInBufLe1/1(LM_OTLCurLeLaObj1Index)
  LM_OTLCurLeLaObj2Index/1 -> LM_OTL_ObjSICNoCurObjInBufLe1/2(LM_OTLCurLeLaObj2Index)
  LM_OTLBufL1LastTPValid/1 -> LM_OTL_ObjSICNoCurObjInBufLe1/10(LM_OTLBufL1LastTPValid)
  LM_OTLBufL1LastEPPos/1 -> LM_OTL_ObjSICNoCurObjInBufLe1/11(LM_OTLBufL1LastEPPos)
  LM_OTLBufDxVectK1Adju/1 -> LM_OTL_ObjSICCurLeObj2InBufLe1/8(LM_OTLBufDxVectK1Adju), LM_OTL_ObjSICCurLeObj1InBufLe1/8(LM_OTLBufDxVectK1Adju)

== system LM_LIB/LM_OTL_Buf2InfoUpdate/LM_OTL_BufLe1InfoUpdate ==
  LM_OTLBufL1DxVectK1Adju : Inport
  LM_OTLBufL1DyVectK1Adju : Inport  Port=2
  LM_OTLBufL1UpdateFlg : Inport  Port=3
  LM_OTLBufL1Objdx : Inport  Port=4
  LM_OTLBufL1Objdy : Inport  Port=5
  LM_OTLBufL1EPPos : Inport  Port=6
  If : If  IfExpression=u1 ~= 0
  If Action Subsystem : Subsystem  TreatAsAtomicUnit=on
  If Action Subsystem1 : Subsystem  TreatAsAtomicUnit=on
  Merge : Merge
  Merge1 : Merge
  LM_OTLBufL1DxVect : Outport  OutDataTypeStr=single  PortDimensions=80
  LM_OTLBufL1DyVect : Outport  Port=2  OutDataTypeStr=single  PortDimensions=80
  wires:
  Merge1/1 -> LM_OTLBufL1DyVect/1  "LM_OTLBufL1DyVect"
  If Action Subsystem1/2(LM_OTLBufL1DyVect) -> Merge1/2
  If Action Subsystem/2(LM_OTLBufL1DyVect) -> Merge1/1
  Merge/1 -> LM_OTLBufL1DxVect/1  "LM_OTLBufL1DxVect"
  If Action Subsystem1/1(LM_OTLBufL1DxVect) -> Merge/2
  If Action Subsystem/1(LM_OTLBufL1DxVect) -> Merge/1
  LM_OTLBufL1EPPos/1 -> If Action Subsystem/3(LM_OTLBufL1EPPos)
  LM_OTLBufL1Objdy/1 -> If Action Subsystem/2(LM_OTLBufL1Objdy)
  LM_OTLBufL1Objdx/1 -> If Action Subsystem/1(LM_OTLBufL1Objdx)
  LM_OTLBufL1DyVectK1Adju/1 -> If Action Subsystem1/2(LM_OTLBufL1DyVectK1Adju), If Action Subsystem/5(LM_OTLBufL1DyVectK1Adju)
  LM_OTLBufL1DxVectK1Adju/1 -> If Action Subsystem1/1(LM_OTLBufL1DxVectK1Adju), If Action Subsystem/4(LM_OTLBufL1DxVectK1Adju)
  If/2 -> If Action Subsystem1/Action
  If/1 -> If Action Subsystem/Action
  LM_OTLBufL1UpdateFlg/1 -> If/1

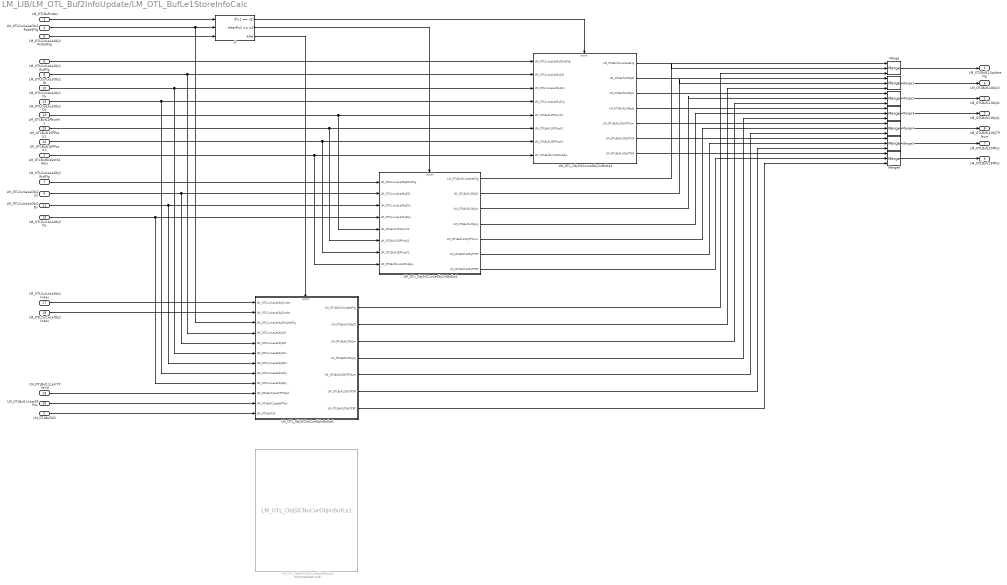
== system LM_LIB/LM_OTL_Buf2InfoUpdate/LM_OTL_BufLe1StoreInfoCalc ==
  LM_OTLBufDxVectK1Adju : Inport
  LM_OTLBuf1ID : Inport  Port=2
  LM_OTLBufIndex : Inport  Port=3
  LM_OTLCurLeLaObj1RcdedFlg : Inport  Port=4
  LM_OTLCurLeLaObj2RcdedFlg : Inport  Port=5
  LM_OTLCurLeLaObj1RcdFlg : Inport  Port=6
  LM_OTLCurLeLaObj2RcdFlg : Inport  Port=7
  LM_OTLCurLeLaObj1ID : Inport  Port=8
  LM_OTLCurLeLaObj2ID : Inport  Port=9
  LM_OTLCurLeLaObj1Dx : Inport  Port=10
  LM_OTLCurLeLaObj2Dx : Inport  Port=11
  LM_OTLCurLeLaObj1Dy : Inport  Port=12
  LM_OTLCurLeLaObj2Dy : Inport  Port=13
  LM_OTLBufL1PNumK1 : Inport  Port=14
  LM_OTLBufL1SPPosK1 : Inport  Port=15
  LM_OTLBufL1EPPosK1 : Inport  Port=16
  LM_OTLCurLeLaObj1Index : Inport  Port=17
  LM_OTLCurLeLaObj2Index : Inport  Port=18
  LM_OTLBufL1LastTPValid : Inport  Port=19
  LM_OTLBufL1LastEPPos : Inport  Port=20
  If : If  NumInputs=3  IfExpression=u1 == u2  ElseIfExpressions=u1 == u3
  LM_OTL_ObjSICCurLeObj1InBufLe1 : Subsystem
  LM_OTL_ObjSICCurLeObj2InBufLe1 : Subsystem
  LM_OTL_ObjSICNoCurObjInBufLe1 : Subsystem
  LM_OTL_ObjSICNoCurObjInBufLe2 : $bdroot/LM_OTL_Buf2InfoUpdate/LM_OTL_BufLe1StoreInfoCalc/LM_OTL_ObjSICNoCurObjInBufLe1  Commented=on  SystemSampleTime=-1  Latency=0  AutoFrameSizeCalculation=off
  Merge{,1..6} (7 alike) : Merge  Inputs=3
  LM_OTLBufL1UpdateFlg : Outport
  LM_OTLBufL1Objdx : Outport  Port=2
  LM_OTLBufL1Objdy : Outport  Port=3
  LM_OTLBufL1EPPos : Outport  Port=4
  LM_OTLBufL1ObjID : Outport  Port=5
  LM_OTLBufL1ObjTPNum : Outport  Port=6
  LM_OTLBufL1SPPos : Outport  Port=7
  wires:
  LM_OTLBufIndex/1 -> If/1
  If/1 -> LM_OTL_ObjSICCurLeObj1InBufLe1/Action
  If/2 -> LM_OTL_ObjSICCurLeObj2InBufLe1/Action
  If/3 -> LM_OTL_ObjSICNoCurObjInBufLe1/Action
  LM_OTLCurLeLaObj1RcdedFlg/1 -> LM_OTL_ObjSICNoCurObjInBufLe1/3(LM_OTLCurLeLaObj1RcdedFlg), If/2
  LM_OTLCurLeLaObj2RcdedFlg/1 -> If/3
  LM_OTLCurLeLaObj1RcdFlg/1 -> LM_OTL_ObjSICCurLeObj1InBufLe1/1(LM_OTLCurLeLaObj1RcdFlg)
  LM_OTLCurLeLaObj1ID/1 -> LM_OTL_ObjSICNoCurObjInBufLe1/4(LM_OTLCurLeLaObj1ID), LM_OTL_ObjSICCurLeObj1InBufLe1/2(LM_OTLCurLeLaObj1ID)
  LM_OTLCurLeLaObj1Dx/1 -> LM_OTL_ObjSICNoCurObjInBufLe1/6(LM_OTLCurLeLaObj1Dx), LM_OTL_ObjSICCurLeObj1InBufLe1/3(LM_OTLCurLeLaObj1Dx)
  LM_OTLCurLeLaObj1Dy/1 -> LM_OTL_ObjSICNoCurObjInBufLe1/8(LM_OTLCurLeLaObj1Dy), LM_OTL_ObjSICCurLeObj1InBufLe1/4(LM_OTLCurLeLaObj1Dy)
  LM_OTLBufL1PNumK1/1 -> LM_OTL_ObjSICCurLeObj2InBufLe1/5(LM_OTLBufL1PNumK1), LM_OTL_ObjSICCurLeObj1InBufLe1/5(LM_OTLBufL1PNumK1)
  LM_OTLBufL1SPPosK1/1 -> LM_OTL_ObjSICCurLeObj2InBufLe1/6(LM_OTLBufL1SPPosK1), LM_OTL_ObjSICCurLeObj1InBufLe1/6(LM_OTLBufL1SPPosK1)
  LM_OTLBufL1EPPosK1/1 -> LM_OTL_ObjSICCurLeObj2InBufLe1/7(LM_OTLBufL1EPPosK1), LM_OTL_ObjSICCurLeObj1InBufLe1/7(LM_OTLBufL1EPPosK1)
  LM_OTLCurLeLaObj2RcdFlg/1 -> LM_OTL_ObjSICCurLeObj2InBufLe1/1(LM_OTLCurLeLaObj2RcdFlg)
  LM_OTLCurLeLaObj2ID/1 -> LM_OTL_ObjSICNoCurObjInBufLe1/5(LM_OTLCurLeLaObj2ID), LM_OTL_ObjSICCurLeObj2InBufLe1/2(LM_OTLCurLeLaObj2ID)
  LM_OTLCurLeLaObj2Dx/1 -> LM_OTL_ObjSICNoCurObjInBufLe1/7(LM_OTLCurLeLaObj2Dx), LM_OTL_ObjSICCurLeObj2InBufLe1/3(LM_OTLCurLeLaObj2Dx)
  LM_OTLCurLeLaObj2Dy/1 -> LM_OTL_ObjSICNoCurObjInBufLe1/9(LM_OTLCurLeLaObj2Dy), LM_OTL_ObjSICCurLeObj2InBufLe1/4(LM_OTLCurLeLaObj2Dy)
  LM_OTL_ObjSICCurLeObj1InBufLe1/1(LM_OTLBufL1UpdateFlg) -> Merge/1
  Merge/1 -> LM_OTLBufL1UpdateFlg/1
  LM_OTL_ObjSICCurLeObj1InBufLe1/2(LM_OTLBufL1ObjID) -> Merge1/1
  Merge1/1 -> LM_OTLBufL1ObjID/1
  LM_OTL_ObjSICCurLeObj1InBufLe1/3(LM_OTLBufL1Objdx) -> Merge2/1
  Merge2/1 -> LM_OTLBufL1Objdx/1
  LM_OTL_ObjSICCurLeObj1InBufLe1/4(LM_OTLBufL1Objdy) -> Merge3/1
  Merge3/1 -> LM_OTLBufL1Objdy/1
  LM_OTL_ObjSICCurLeObj1InBufLe1/5(LM_OTLBufL1ObjTPNum) -> Merge4/1
  Merge4/1 -> LM_OTLBufL1ObjTPNum/1
  LM_OTL_ObjSICCurLeObj1InBufLe1/6(LM_OTLBufL1ObjTPSP) -> Merge5/1
  Merge5/1 -> LM_OTLBufL1SPPos/1
  LM_OTL_ObjSICCurLeObj1InBufLe1/7(LM_OTLBufL1ObjTPEP) -> Merge6/1
  Merge6/1 -> LM_OTLBufL1EPPos/1
  LM_OTL_ObjSICCurLeObj2InBufLe1/1(LM_OTLBufL1UpdateFlg) -> Merge/2
  LM_OTL_ObjSICCurLeObj2InBufLe1/2(LM_OTLBufL1ObjID) -> Merge1/2
  LM_OTL_ObjSICCurLeObj2InBufLe1/3(LM_OTLBufL1Objdx) -> Merge2/2
  LM_OTL_ObjSICCurLeObj2InBufLe1/4(LM_OTLBufL1Objdy) -> Merge3/2
  LM_OTL_ObjSICCurLeObj2InBufLe1/5(LM_OTLBufL1ObjTPNum) -> Merge4/2
  LM_OTL_ObjSICCurLeObj2InBufLe1/6(LM_OTLBufL1ObjTPSP) -> Merge5/2
  LM_OTL_ObjSICCurLeObj2InBufLe1/7(LM_OTLBufL1ObjTPEP) -> Merge6/2
  LM_OTL_ObjSICNoCurObjInBufLe1/1(LM_OTLBufL2UpdateFlg) -> Merge/3
  LM_OTL_ObjSICNoCurObjInBufLe1/2(LM_OTLBufL2ObjID) -> Merge1/3
  LM_OTL_ObjSICNoCurObjInBufLe1/3(LM_OTLBufL2Objdx) -> Merge2/3
  LM_OTL_ObjSICNoCurObjInBufLe1/4(LM_OTLBufL2Objdy) -> Merge3/3
  LM_OTL_ObjSICNoCurObjInBufLe1/5(LM_OTLBufL2ObjTPNum) -> Merge4/3
  LM_OTL_ObjSICNoCurObjInBufLe1/6(LM_OTLBufL2ObjTPSP) -> Merge5/3
  LM_OTL_ObjSICNoCurObjInBufLe1/7(LM_OTLBufL2ObjTPEP) -> Merge6/3
  LM_OTLCurLeLaObj1Index/1 -> LM_OTL_ObjSICNoCurObjInBufLe1/1(LM_OTLCurLeLaObj1Index)
  LM_OTLCurLeLaObj2Index/1 -> LM_OTL_ObjSICNoCurObjInBufLe1/2(LM_OTLCurLeLaObj2Index)
  LM_OTLBufL1LastTPValid/1 -> LM_OTL_ObjSICNoCurObjInBufLe1/10(LM_OTLBufL1LastTPValid)
  LM_OTLBufL1LastEPPos/1 -> LM_OTL_ObjSICNoCurObjInBufLe1/11(LM_OTLBufL1LastEPPos)
  LM_OTLBuf1ID/1 -> LM_OTL_ObjSICNoCurObjInBufLe1/12(LM_OTLBuf1ID)
  LM_OTLBufDxVectK1Adju/1 -> LM_OTL_ObjSICCurLeObj2InBufLe1/8(LM_OTLBufDxVectK1Adju), LM_OTL_ObjSICCurLeObj1InBufLe1/8(LM_OTLBufDxVectK1Adju)

== system LM_LIB/LM_OTL_BufTPInfoEva/LM_OTL_BufLe1TPInfoCalc ==
  LM_OTLBufUsefulTPObjFlg : Inport
  LM_OTLBufL1PNum : Inport  Port=2
  LM_OTLBufL1SPPos : Inport  Port=3
  LM_OTLBufL1EPPos : Inport  Port=4
  LM_OTLBufL1LastSPPos : Inport  Port=5
  LM_OTLBufL1LastEPPos : Inport  Port=6
  LM_OTLBufL1LastPNum : Inport  Port=7
  Constant : Constant  OutDataTypeStr=uint8
  Constant1 : Constant  Value=2  OutDataTypeStr=uint8
  Constant2 : Constant  Value=0  OutDataTypeStr=uint8
  Relational Operator : RelationalOperator  Operator===  OutDataTypeStr=boolean  RndMeth=Simplest
  Relational Operator1 : RelationalOperator  Operator===  OutDataTypeStr=boolean  RndMeth=Simplest
  Switch{,1..5} (6 alike) : Switch  Criteria=u2 ~= 0
  LM_OTLBufL1ValidTPNum : Outport
  LM_OTLBufL1ValidSPPos : Outport  Port=2
  LM_OTLBufL1ValidEPPos : Outport  Port=3
  wires:
  Switch4/1 -> LM_OTLBufL1ValidEPPos/1  "LM_OTLBufL1ValidEPPos"
  LM_OTLBufL1LastEPPos/1 -> Switch5/1
  Switch5/1 -> Switch4/3
  LM_OTLBufL1EPPos/1 -> Switch4/1
  Switch2/1 -> LM_OTLBufL1ValidSPPos/1  "LM_OTLBufL1ValidSPPos"
  Switch3/1 -> Switch2/3
  LM_OTLBufL1LastSPPos/1 -> Switch3/1
  LM_OTLBufL1SPPos/1 -> Switch2/1
  Constant2/1 -> Switch1/3, Switch3/3, Switch5/3
  Switch1/1 -> Switch/3
  LM_OTLBufL1LastPNum/1 -> Switch1/1
  Relational Operator1/1 -> Switch1/2, Switch3/2, Switch5/2
  Constant1/1 -> Relational Operator1/2
  Switch/1 -> LM_OTLBufL1ValidTPNum/1  "LM_OTLBufL1ValidTPNum"
  LM_OTLBufL1PNum/1 -> Switch/1
  Relational Operator/1 -> Switch/2, Switch2/2, Switch4/2
  Constant/1 -> Relational Operator/2
  LM_OTLBufUsefulTPObjFlg/1 -> Relational Operator/1, Relational Operator1/1

== system LM_LIB/LM_OTL_BufTPInfoEva/LM_OTL_BufLe1TPPosInfo ==
  LM_OTLBufL1DxVect : Inport
  LM_OTLBufL1DyVect : Inport  Port=2
  LM_OTLBufL1PNum : Inport  Port=3
  LM_OTLBufL1SPPos : Inport  Port=4
  LM_OTLBufL1EPPos : Inport  Port=5
  LM_OTLBufL1LastTPValid : Inport  Port=6
  LM_OTLBufL1LastSPPos : Inport  Port=7
  LM_OTLBufL1LastEPPos : Inport  Port=8
  Compare To Zero{,1..3} (4 alike) : simulink/Logic and Bit Operations/Compare To Zero  relop===  OutDataTypeStr=boolean
  Constant : Constant  Value=0  OutDataTypeStr=single
  Constant1 : Constant  OutDataTypeStr=uint8
  Constant2 : Constant  Value=0  OutDataTypeStr=single
  Constant3 : Constant  OutDataTypeStr=uint8
  Index Vector{,1..3} (4 alike) : MultiPortSwitch  Inputs=1
  Switch{,1..7} (8 alike) : Switch  Criteria=u2 ~= 0
  Terminator : Terminator
  Terminator1 : Terminator
  LM_OTLBufLe1CSOdxStart : Outport
  LM_OTLBufLe1LSOdxStart : Outport  Port=2
  wires:
  Switch5/1 -> Terminator/1  "LM_OTLBufLe1LSOdxEnd"
  Switch4/1 -> LM_OTLBufLe1LSOdxStart/1  "LM_OTLBufLe1LSOdxStart"
  Index Vector3/1 -> Switch5/3
  Index Vector2/1 -> Switch4/3
  Switch7/1 -> Index Vector3/1
  Switch6/1 -> Index Vector2/1
  Compare To Zero1/1 -> Switch4/2, Switch5/2
  Constant3/1 -> Switch7/1, Switch6/1
  LM_OTLBufL1LastSPPos/1 -> Switch6/3, Compare To Zero2/1
  LM_OTLBufL1LastEPPos/1 -> Switch7/3, Compare To Zero3/1
  Constant2/1 -> Switch4/1, Switch5/1
  LM_OTLBufL1LastTPValid/1 -> Compare To Zero1/1
  Switch3/1 -> Terminator1/1  "LM_OTLBufLe1CSOdxEnd"
  Index Vector1/1 -> Switch3/3
  LM_OTLBufL1DyVect/1 -> Index Vector1/2, Index Vector3/2
  Switch2/1 -> Index Vector1/1
  Switch/1 -> LM_OTLBufLe1CSOdxStart/1  "LM_OTLBufLe1CSOdxStart"
  Index Vector/1 -> Switch/3
  Switch1/1 -> Index Vector/1
  LM_OTLBufL1DxVect/1 -> Index Vector/2, Index Vector2/2
  LM_OTLBufL1EPPos/1 -> Switch2/3
  LM_OTLBufL1SPPos/1 -> Switch1/3
  Constant1/1 -> Switch1/1, Switch2/1
  Constant/1 -> Switch/1, Switch3/1
  Compare To Zero/1 -> Switch/2, Switch3/2, Switch1/2, Switch2/2
  LM_OTLBufL1PNum/1 -> Compare To Zero/1
  Compare To Zero2/1 -> Switch6/2
  Compare To Zero3/1 -> Switch7/2

== system LM_LIB/LM_OTL_BufTPInfoEva/LM_OTL_BufLe1UsefulObjTPSelc ==
  note: P_LM_OTLBufTPMinPntNum
  note: P_LM_OTLBufTPSPosMinDis
  note: 0:轨迹点存储buffer中无可利用的轨迹点信息
      | 1:轨迹点存储buffer中当前存储目标轨迹点可利用
      | 2:轨迹点存储buffer中上一存储目标轨迹点可利用
  LM_OTLBufLe1CSOdxStart : Inport
  LM_OTLBufLe1LSOdxStart : Inport  Port=2
  LM_OTLBufL1PNum : Inport  Port=3
  LM_OTLBufL1LastTPValid : Inport  Port=4
  LM_OTLBufL1LastPNum : Inport  Port=5
  Compare To Zero : simulink/Logic and Bit Operations/Compare To Zero  relop=~=  OutDataTypeStr=boolean
  Constant : Constant  Value=P_LM_OTLBufTPMinPntNum
  Constant1 : Constant  Value=P_LM_OTLBufTPSPosMinDis
  Constant2 : Constant  OutDataTypeStr=uint8
  Constant3 : Constant  Value=0  OutDataTypeStr=uint8
  Constant4 : Constant  Value=2  OutDataTypeStr=uint8
  DocBlock : simulink/Model-Wide Utilities/DocBlock  DocumentType=Text
      content=|
      | Type your documentation here
  Logical Operator : Logic  AllPortsSameDT=off  OutDataTypeStr=boolean
  Logical Operator1 : Logic  AllPortsSameDT=off  OutDataTypeStr=boolean
  Relational Operator : RelationalOperator  OutDataTypeStr=boolean  RndMeth=Simplest
  Relational Operator1 : RelationalOperator  Operator=<=  OutDataTypeStr=boolean  RndMeth=Simplest
  Relational Operator2 : RelationalOperator  OutDataTypeStr=boolean  RndMeth=Simplest
  Relational Operator3 : RelationalOperator  Operator=<=  OutDataTypeStr=boolean  RndMeth=Simplest
  Switch : Switch  Criteria=u2 ~= 0
  Switch1 : Switch  Criteria=u2 ~= 0
  Switch2 : Switch  Criteria=u2 ~= 0
  LM_OTLBufUsefulTPObjFlg : Outport
  wires:
  Switch/1 -> LM_OTLBufUsefulTPObjFlg/1  "LM_OTLBufUsefulTPObjFlg"
  Switch1/1 -> Switch/3
  Switch2/1 -> Switch1/1
  Constant4/1 -> Switch2/1
  Logical Operator1/1 -> Switch2/2
  Relational Operator3/1 -> Logical Operator1/2
  Relational Operator2/1 -> Logical Operator1/1
  LM_OTLBufLe1LSOdxStart/1 -> Relational Operator3/1
  LM_OTLBufL1LastPNum/1 -> Relational Operator2/1
  Constant3/1 -> Switch2/3, Switch1/3
  Compare To Zero/1 -> Switch1/2
  LM_OTLBufL1LastTPValid/1 -> Compare To Zero/1
  Constant2/1 -> Switch/1
  Logical Operator/1 -> Switch/2
  Relational Operator1/1 -> Logical Operator/2
  Constant1/1 -> Relational Operator1/2, Relational Operator3/2
  LM_OTLBufLe1CSOdxStart/1 -> Relational Operator1/1
  Relational Operator/1 -> Logical Operator/1
  Constant/1 -> Relational Operator/2, Relational Operator2/2
  LM_OTLBufL1PNum/1 -> Relational Operator/1

== system LM_LIB/LM_LineInfo1/LM_Line_Fnt/LM_Path04 ==
  LM_FusBLFntPath1C0 : Inport
  LM_FusBLFntPath1C1 : Inport  Port=2
  LM_FusBLFntPath1C2 : Inport  Port=3
  LM_FusBLFntPath1C3 : Inport  Port=4
  LM_FusBLFntPath1Quality : Inport  Port=5
  LM_LineC0 : Inport  Port=6
  LM_FusFntPath1Dis : Inport  Port=7
  LM_FusFntPath1fCamValid : Inport  Port=8
  Add : Sum
  Bus Creator : BusCreator  Inputs=8  OutDataTypeStr=Bus: LM_TRAJINFO_BUS  NonVirtualBus=on
  Compare To Zero : simulink/Logic and Bit Operations/Compare To Zero  relop===  OutDataTypeStr=boolean
  Constant : Constant  Value=0  OutDataTypeStr=single
  Signal Conversion{,1..7} (8 alike) : SignalConversion  OverrideOpt=off
  Switch : Switch  Criteria=u2 ~= 0
  Switch1 : Switch  Criteria=u2 ~= 0
  Switch2 : Switch  Criteria=u2 ~= 0
  LM_Line04 : Outport
  wires:
  Add/1 -> Switch2/3
  LM_FusBLFntPath1C0/1 -> Add/1
  Switch2/1 -> Signal Conversion/1
  Switch1/1 -> Signal Conversion5/1
  Compare To Zero/1 -> Switch/2, Switch2/2, Switch1/2
  Switch/1 -> Signal Conversion6/1
  Signal Conversion7/1 -> Bus Creator/8  "fCamValid"
  Signal Conversion6/1 -> Bus Creator/7  "dQuality"
  Signal Conversion5/1 -> Bus Creator/6  "dDisEnd"
  Signal Conversion4/1 -> Bus Creator/5  "dDisStart"
  Signal Conversion3/1 -> Bus Creator/4  "pC3"
  Signal Conversion2/1 -> Bus Creator/3  "pC2"
  Signal Conversion1/1 -> Bus Creator/2  "pC1"
  Signal Conversion/1 -> Bus Creator/1  "pC0"
  Bus Creator/1 -> LM_Line04/1  "LM_Line04"
  LM_FusFntPath1fCamValid/1 -> Signal Conversion7/1
  LM_FusBLFntPath1Quality/1 -> Compare To Zero/1, Switch/3
  Constant/1 -> Signal Conversion4/1, Switch1/1, Switch/1, Switch2/1
  LM_FusFntPath1Dis/1 -> Switch1/3
  LM_FusBLFntPath1C3/1 -> Signal Conversion3/1
  LM_FusBLFntPath1C2/1 -> Signal Conversion2/1
  LM_FusBLFntPath1C1/1 -> Signal Conversion1/1
  LM_LineC0/1 -> Add/2
